simulink model "scars_sentinel"  (R2019b)
settings: Solver=ode14x  StartTime=0.0  StopTime=1  FixedStep=0.0025  MaxStep=1  MinStep=dT  RelTol=1e-3
model workspace (MAT data in the model file):
  actuators = 0
  delay = 1
  displacement = 1
  i_max = 1
  torq_max = 1
  vel_max = 1
libraries: scars_library x31
settings Model: OrderedModelArguments=off  Creator=asmialek  LastModifiedBy=asmialek
settings DataIOCC: SaveFormat=Array  ReturnWorkspaceOutputsName=scars_out

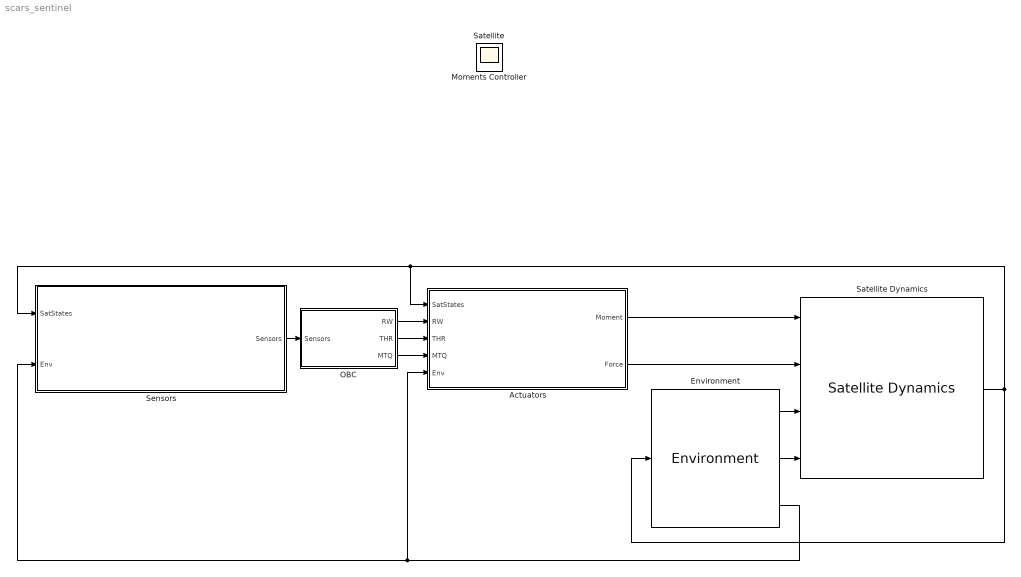
== system scars_sentinel ==
  Actuators : Subsystem
  Environment : scars_library/Environment/Environment  SystemSampleTime=-1  Latency=0  AutoFrameSizeCalculation=off
  OBC : Subsystem
  Satellite Dynamics : scars_library/Advanced/Satellite Dynamics  Parameter4=Keplerian Elements  epoch=0  mass=0  a=6356e3+400e3  e=0  incl=0  RA=0  w=0  TA=0  initEuler=[0 0 0]  initEulerRates=[0 0 0]  TA_copy=0  TA_copy_copy=400e3  TA_copy_copy_copy=[10 25]  TA_copy_copy_copy_copy=[10 25]  initEuler_copy=[0 0 0]  initEulerRates_copy=[0 0 0]  mask(Sattellite Dynamics){}
      mask Display: image('C:\master_thesis\scars_toolbox\resources\sentinel.jpg'); % Use "Edit Image" on toolstrip to change.
  Sensors : Subsystem
  Moments Controller : Scope
  Satellite : Scope
  wires:
  Environment/1 -> Satellite Dynamics/3
  Environment/2 -> Satellite Dynamics/4
  Environment/3 -> Sensors/2("Env "), Actuators/5(Env)
  Actuators/1(Moment) -> Satellite Dynamics/1
  Actuators/2(Force) -> Satellite Dynamics/2
  Satellite Dynamics/1 -> Environment/1, Sensors/1("SatStates "), Actuators/1(SatStates)
  OBC/1(RW) -> Actuators/2(RW)
  OBC/2(THR) -> Actuators/3(THR)
  OBC/3(MTQ) -> Actuators/4(MTQ)
  Sensors/1(Sensors) -> OBC/1(Sensors)

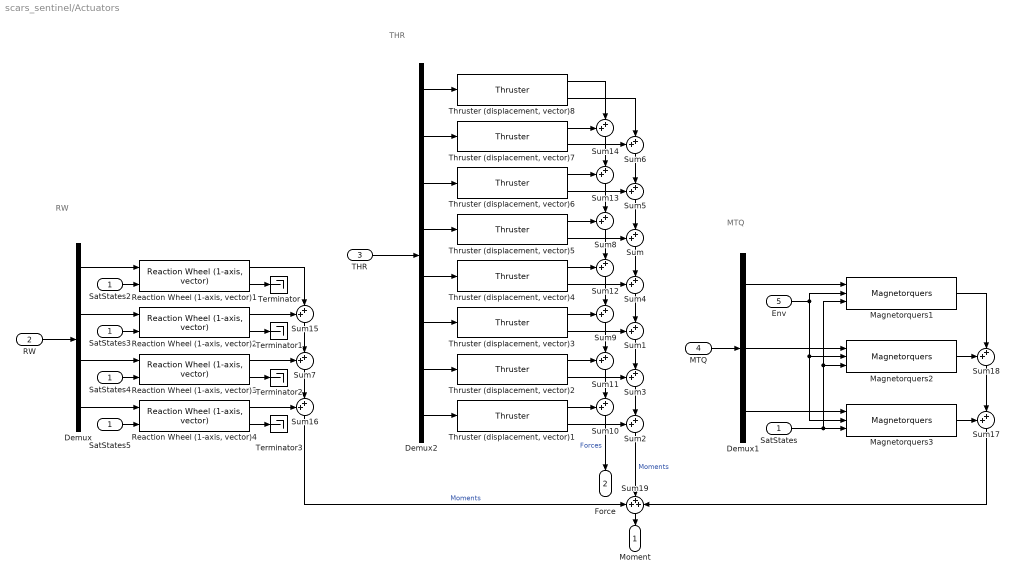
== system scars_sentinel/Actuators ==
  note: MTQ
  note: RW
  note: THR
  SatStates : Inport
  RW : Inport  Port=2
  THR : Inport  Port=3
  MTQ : Inport  Port=4
  Env : Inport  Port=5
  Demux : Demux
  Demux1 : Demux  Outputs=3
  Demux2 : Demux  Outputs=8
  Magnetorquers1 : scars_library/Actuators/Magnetorquers  L_mt=2.666  R_mt=3.621  l_c_mt=0.25  w_c_mt=7.965e-3  d_w_mt=4.04e-4  mag_vol_max=3  mag_vol_min=-3
  Magnetorquers2 : scars_library/Actuators/Magnetorquers  L_mt=2.666  R_mt=3.621  l_c_mt=0.25  w_c_mt=7.965e-3  d_w_mt=4.04e-4  mag_vol_max=3  mag_vol_min=-3
  Magnetorquers3 : scars_library/Actuators/Magnetorquers  L_mt=2.666  R_mt=3.621  l_c_mt=0.25  w_c_mt=7.965e-3  d_w_mt=4.04e-4  mag_vol_max=3  mag_vol_min=-3
  Reaction Wheel (1-axis, vector){1..4} (4 alike) : scars_library/Actuators/Reaction Wheel (1-axis, vector)  op_vec=[1 0 0]  N=25e-3  R=0.1  J=1  c=0.0001  rw_power=0.0001  rw_freq=0.1
  SatStates{2..5} (4 alike) : InportShadow
  Sum{,1..18} (19 alike) : Sum  Inputs=++|
  Sum19 : Sum  Inputs=+++
  Terminator{,1..3} (4 alike) : Terminator
  Thruster (displacement, vector){1..8} (8 alike) : scars_library/Actuators/Thruster  SystemSampleTime=-1  Latency=0  AutoFrameSizeCalculation=off
  Moment : Outport
  Force : Outport  Port=2
  wires:
  Demux2/1 -> "Thruster (displacement, vector)8"/1
  "Reaction Wheel (1-axis, vector)4"/1 -> Sum16/1
  Sum15/1 -> Sum7/2
  Demux/4 -> "Reaction Wheel (1-axis, vector)4"/1
  "Thruster (displacement, vector)2"/2 -> Sum3/1
  "Thruster (displacement, vector)2"/1 -> Sum11/1
  "Thruster (displacement, vector)3"/2 -> Sum1/1
  Sum6/1 -> Sum5/2
  "Thruster (displacement, vector)6"/2 -> Sum5/1
  "Reaction Wheel (1-axis, vector)4"/2 -> Terminator3/1
  Demux2/3 -> "Thruster (displacement, vector)6"/1
  Sum13/1 -> Sum8/2
  Demux1/3 -> Magnetorquers3/1
  Sum11/1 -> Sum10/2
  Sum14/1 -> Sum13/2
  "Thruster (displacement, vector)7"/2 -> Sum6/1
  Sum/1 -> Sum4/2
  Sum9/1 -> Sum11/2
  Sum8/1 -> Sum12/2
  "Thruster (displacement, vector)7"/1 -> Sum14/1
  Demux1/2 -> Magnetorquers2/1
  Sum2/1 -> Sum19/2  "Moments"
  Demux2/5 -> "Thruster (displacement, vector)4"/1
  Demux1/1 -> Magnetorquers1/1
  "Thruster (displacement, vector)4"/2 -> Sum4/1
  Sum4/1 -> Sum1/2
  "Reaction Wheel (1-axis, vector)2"/1 -> Sum15/1
  Env/1 -> Magnetorquers1/2, Magnetorquers3/2, Magnetorquers2/2
  Demux/2 -> "Reaction Wheel (1-axis, vector)2"/1
  Sum10/1 -> Force/1  "Forces"
  Sum16/1 -> Sum19/1  "Moments"
  Demux2/2 -> "Thruster (displacement, vector)7"/1
  SatStates/1 -> Magnetorquers1/3, Magnetorquers2/3, Magnetorquers3/3
  "Reaction Wheel (1-axis, vector)1"/2 -> Terminator/1
  "Reaction Wheel (1-axis, vector)3"/2 -> Terminator2/1
  Sum5/1 -> Sum/2
  "Reaction Wheel (1-axis, vector)2"/2 -> Terminator1/1
  Demux2/8 -> "Thruster (displacement, vector)1"/1
  "Thruster (displacement, vector)8"/2 -> Sum6/2
  SatStates3/1 -> "Reaction Wheel (1-axis, vector)2"/2
  SatStates5/1 -> "Reaction Wheel (1-axis, vector)4"/2
  Demux/3 -> "Reaction Wheel (1-axis, vector)3"/1
  SatStates4/1 -> "Reaction Wheel (1-axis, vector)3"/2
  Demux2/7 -> "Thruster (displacement, vector)2"/1
  Demux2/6 -> "Thruster (displacement, vector)3"/1
  Demux/1 -> "Reaction Wheel (1-axis, vector)1"/1
  Sum1/1 -> Sum3/2
  "Reaction Wheel (1-axis, vector)1"/1 -> Sum15/2
  "Thruster (displacement, vector)4"/1 -> Sum12/1
  Demux2/4 -> "Thruster (displacement, vector)5"/1
  Sum7/1 -> Sum16/2
  "Thruster (displacement, vector)6"/1 -> Sum13/1
  "Thruster (displacement, vector)1"/2 -> Sum2/1
  "Thruster (displacement, vector)1"/1 -> Sum10/1
  "Thruster (displacement, vector)5"/2 -> Sum/1
  Sum3/1 -> Sum2/2
  "Reaction Wheel (1-axis, vector)3"/1 -> Sum7/1
  SatStates2/1 -> "Reaction Wheel (1-axis, vector)1"/2
  "Thruster (displacement, vector)5"/1 -> Sum8/1
  "Thruster (displacement, vector)8"/1 -> Sum14/2
  Sum12/1 -> Sum9/2
  "Thruster (displacement, vector)3"/1 -> Sum9/1
  Sum18/1 -> Sum17/2
  Sum17/1 -> Sum19/3
  Magnetorquers1/1 -> Sum18/2
  Magnetorquers2/1 -> Sum18/1
  Magnetorquers3/1 -> Sum17/1
  Sum19/1 -> Moment/1
  RW/1 -> Demux/1
  THR/1 -> Demux2/1
  MTQ/1 -> Demux1/1

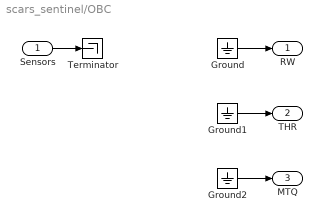
== system scars_sentinel/OBC ==
  Sensors : Inport
  Ground : Ground
  Ground1 : Ground
  Ground2 : Ground
  Terminator : Terminator
  RW : Outport
  THR : Outport  Port=2
  MTQ : Outport  Port=3
  wires:
  Sensors/1 -> Terminator/1
  Ground/1 -> RW/1
  Ground1/1 -> THR/1
  Ground2/1 -> MTQ/1

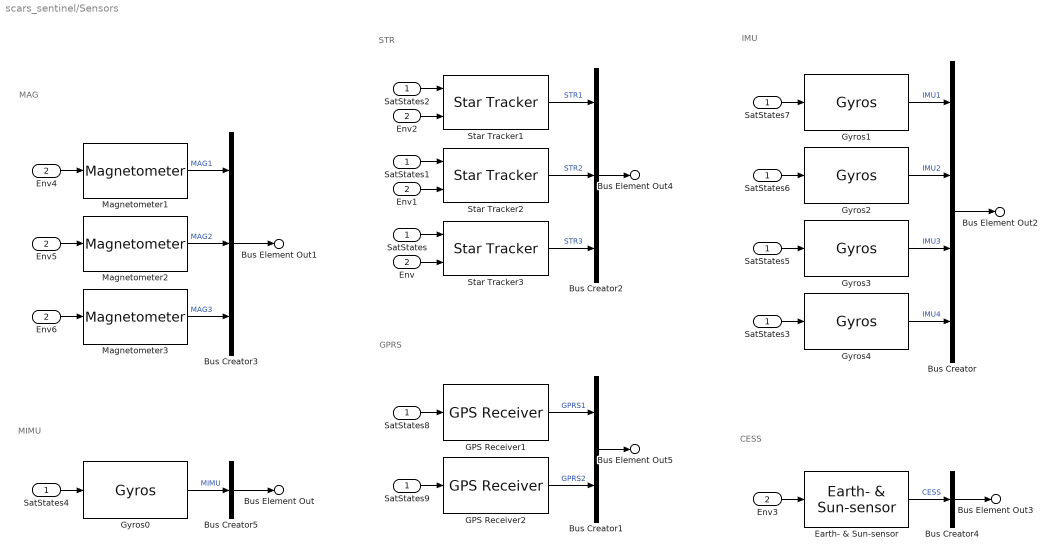
== system scars_sentinel/Sensors ==
  note: MIMU
  note: MAG
  note: CESS
  note: IMU
  note: GPRS
  note: STR
  "SatStates " : Inport
  "Env " : Inport  Port=2
  Bus Creator : BusCreator  Inputs=4
  Bus Creator1 : BusCreator  Inputs=2
  Bus Creator2 : BusCreator  Inputs=3
  Bus Creator3 : BusCreator  Inputs=3
  Bus Creator4 : BusCreator  Inputs=1
  Bus Creator5 : BusCreator  Inputs=1
  Earth- & Sun-sensor : scars_library/Sensors/Earth- & Sun-sensor  SystemSampleTime=-1  Latency=0  AutoFrameSizeCalculation=off
  Env{1..6} (6 alike) : InportShadow  Port=2
  GPS Receiver1 : scars_library/Sensors/GPS Receiver  SystemSampleTime=-1  Latency=0  AutoFrameSizeCalculation=off
  GPS Receiver2 : scars_library/Sensors/GPS Receiver  SystemSampleTime=-1  Latency=0  AutoFrameSizeCalculation=off
  Gyros{0..4} (5 alike) : scars_library/Sensors/Gyros  g_wn=1000*2*pi  g_zeta=sqrt(2)/2  g_freq=80  g_bias=0  g_power=(0.04)^2  g_max=deg2rad(100)  g_min=-deg2rad(100)
  Magnetometer1 : scars_library/Sensors/Magnetometer  m_power=0.1  m_freq=10  m_bias=[0.01 0.01 0.01]
  Magnetometer2 : scars_library/Sensors/Magnetometer  m_power=0.1  m_freq=10  m_bias=[0.01 0.01 0.01]
  Magnetometer3 : scars_library/Sensors/Magnetometer  m_power=0.1  m_freq=10  m_bias=[0.01 0.01 0.01]
  SatStates{1..9} (9 alike) : InportShadow
  Star Tracker1 : scars_library/Sensors/Star Tracker  st_vector=[0 0 -1]  st_ex_sun=20  st_ex_earth=20  st_lost=5  Parameter5=10
  Star Tracker2 : scars_library/Sensors/Star Tracker  st_vector=[0 0 -1]  st_ex_sun=20  st_ex_earth=20  st_lost=5  Parameter5=10
  Star Tracker3 : scars_library/Sensors/Star Tracker  st_vector=[0 0 -1]  st_ex_sun=20  st_ex_earth=20  st_lost=5  Parameter5=10
  Bus Element Out : Outport  PortName=Sensors  Element=MIMU
  Bus Element Out1 : Outport  PortName=Sensors  Element=MAG
  Bus Element Out2 : Outport  PortName=Sensors  Element=IMU
  Bus Element Out3 : Outport  PortName=Sensors  Element=CESS
  Bus Element Out4 : Outport  PortName=Sensors  Element=STR
  Bus Element Out5 : Outport  PortName=Sensors  Element=GPRS
  wires:
  Env1/1 -> Star Tracker2/2
  Star Tracker1/1 -> Bus Creator2/1  "STR1"
  SatStates1/1 -> Star Tracker2/1
  Star Tracker2/1 -> Bus Creator2/2  "STR2"
  Env2/1 -> Star Tracker1/2
  "Env "/1 -> Star Tracker3/2
  "SatStates "/1 -> Star Tracker3/1
  Star Tracker3/1 -> Bus Creator2/3  "STR3"
  SatStates2/1 -> Star Tracker1/1
  Env5/1 -> Magnetometer2/1
  Env4/1 -> Magnetometer1/1
  Magnetometer1/1 -> Bus Creator3/1  "MAG1"
  Env6/1 -> Magnetometer3/1
  Magnetometer2/1 -> Bus Creator3/2  "MAG2"
  SatStates8/1 -> GPS Receiver1/1
  Env3/1 -> Earth- & Sun-sensor/1
  SatStates9/1 -> GPS Receiver2/1
  GPS Receiver2/1 -> Bus Creator1/2  "GPRS2"
  Magnetometer3/1 -> Bus Creator3/3  "MAG3"
  Earth- & Sun-sensor/1 -> Bus Creator4/1  "CESS"
  GPS Receiver1/1 -> Bus Creator1/1  "GPRS1"
  SatStates3/1 -> Gyros4/1
  Gyros3/1 -> Bus Creator/3  "IMU3"
  Gyros4/1 -> Bus Creator/4  "IMU4"
  Gyros1/1 -> Bus Creator/1  "IMU1"
  Gyros2/1 -> Bus Creator/2  "IMU2"
  SatStates4/1 -> Gyros0/1
  Gyros0/1 -> Bus Creator5/1  "MIMU"
  SatStates6/1 -> Gyros2/1
  SatStates7/1 -> Gyros1/1
  SatStates5/1 -> Gyros3/1
  Bus Creator5/1 -> Bus Element Out/1
  Bus Creator3/1 -> Bus Element Out1/1
  Bus Creator/1 -> Bus Element Out2/1
  Bus Creator4/1 -> Bus Element Out3/1
  Bus Creator2/1 -> Bus Element Out4/1
  Bus Creator1/1 -> Bus Element Out5/1
